simulink model "RALFMain"  (R2020a)
settings: Solver=FixedStepAuto  StartTime=0.0  StopTime=inf  FixedStep=0.01  RelTol=1e-3
InitFcn:
  | init
StopFcn:
  | stop
model workspace (MAT data in the model file):
  SL_ROS_VariableLengthArrays_MaxSizes.CommonInfo.ArrayTruncateAction = 'EmitWarning'
  SL_ROS_VariableLengthArrays_MaxSizes.MsgTypeMap = containers.Map
  SL_ROS_VariableLengthArrays_MaxSizes.MsgTypeMap.serialization.keys = {'sensor_msgs/Joy', 'std_msgs/Float32MultiArray', 'std_msgs/Int16MultiArray', 'std_msgs/Int32MultiArray', 'std_msgs/UInt16MultiArray', 'std_msgs/UInt8MultiArray'}
  SL_ROS_VariableLengthArrays_MaxSizes.MsgTypeMap.serialization.values{1}(1).PropertyName = 'Axes'
  SL_ROS_VariableLengthArrays_MaxSizes.MsgTypeMap.serialization.values{1}(1).DataType = 'single'
  SL_ROS_VariableLengthArrays_MaxSizes.MsgTypeMap.serialization.values{1}(1).MaxLength = 8
  SL_ROS_VariableLengthArrays_MaxSizes.MsgTypeMap.serialization.values{1}(2).PropertyName = 'Buttons'
  SL_ROS_VariableLengthArrays_MaxSizes.MsgTypeMap.serialization.values{1}(2).DataType = 'int32'
  SL_ROS_VariableLengthArrays_MaxSizes.MsgTypeMap.serialization.values{1}(2).MaxLength = 15
  SL_ROS_VariableLengthArrays_MaxSizes.MsgTypeMap.serialization.values{2}.PropertyName = 'Data'
  SL_ROS_VariableLengthArrays_MaxSizes.MsgTypeMap.serialization.values{2}.DataType = 'single'
  SL_ROS_VariableLengthArrays_MaxSizes.MsgTypeMap.serialization.values{2}.MaxLength = 8
  SL_ROS_VariableLengthArrays_MaxSizes.MsgTypeMap.serialization.values{3}.PropertyName = 'Data'
  SL_ROS_VariableLengthArrays_MaxSizes.MsgTypeMap.serialization.values{3}.DataType = 'int16'
  SL_ROS_VariableLengthArrays_MaxSizes.MsgTypeMap.serialization.values{3}.MaxLength = 4
  SL_ROS_VariableLengthArrays_MaxSizes.MsgTypeMap.serialization.values{4}.PropertyName = 'Data'
  SL_ROS_VariableLengthArrays_MaxSizes.MsgTypeMap.serialization.values{4}.DataType = 'int32'
  SL_ROS_VariableLengthArrays_MaxSizes.MsgTypeMap.serialization.values{4}.MaxLength = 8
  SL_ROS_VariableLengthArrays_MaxSizes.MsgTypeMap.serialization.values{5}.PropertyName = 'Data'
  SL_ROS_VariableLengthArrays_MaxSizes.MsgTypeMap.serialization.values{5}.DataType = 'uint16'
  SL_ROS_VariableLengthArrays_MaxSizes.MsgTypeMap.serialization.values{5}.MaxLength = 8
  SL_ROS_VariableLengthArrays_MaxSizes.MsgTypeMap.serialization.values{6}.PropertyName = 'Data'
  SL_ROS_VariableLengthArrays_MaxSizes.MsgTypeMap.serialization.values{6}.DataType = 'uint8'
  SL_ROS_VariableLengthArrays_MaxSizes.MsgTypeMap.serialization.values{6}.MaxLength = 8
  SL_ROS_VariableLengthArrays_MaxSizes.MsgTypeMap.serialization.uniformity = 0
  SL_ROS_VariableLengthArrays_MaxSizes.MsgTypeMap.serialization.keyType = 'char'
  SL_ROS_VariableLengthArrays_MaxSizes.MsgTypeMap.serialization.valueType = 'any'
values from neighbouring files (symbols this model uses):
  nmax = 1000    [init.m]
  pwinkel = 1/20    (= 0.05)    [init.m]
  pwinkel_vel = -4    [init.m]
undefined symbols (not defined in the file or in its folder): Axes, Axes_SL_Info, Buttons, Buttons_SL_Info
libraries: simulink x13, robotlib x4, dspswit3 x4, robotcorelib x4, simulink_extras x3, aerolibutil x3, etargetslib x2, aerolibanimutils x1, sharedtransform x1
CloseFcn:
  | stop
settings Model: EnablePacing=on  Creator=alf  LastModifiedBy=alf
settings DataIOCC: ReturnWorkspaceOutputs=off
settings OptimizationCC: EnhancedBackFolding=on  PassReuseOutputArgsAs=Individual arguments  MaxStackSize=64  OptimizeBlockOrder=speed  DifferentSizesBufferReuse=on  OptimizationCustomize=off  EfficientTunableParamExpr=on
settings DebuggingCC: ParameterPrecisionLossMsg=none  ParameterTunabilityLossMsg=error  ArithmeticOperatorsInVariantConditions=warning
settings HardwareCC: ProdBitPerLong=64  ProdHWDeviceType=Intel->x86-64 (Linux 64)
settings SFSimCC: MATLABDynamicMemAlloc=off  CustomCodeUndefinedFunction=UseInterfaceOnly
settings RTWCC: SystemTargetFile=ert.tlc  HardwareBoard=Robot Operating System (ROS)  TemplateMakefile=ert_default_tmf  GenerateReport=on  Toolchain=Catkin  IncludeHyperlinkInReport=on  LaunchReport=on  TargetLang=C++  GenerateTraceInfo=on  GenerateTraceReport=on  GenerateTraceReportSl=on  GenerateTraceReportSf=on  GenerateTraceReportEml=on
settings CodeAppCC: ForceParamTrailComments=on  IgnoreCustomStorageClasses=off  OperatorAnnotations=on  SimulinkDataObjDesc=on  SFDataObjDesc=on  InsertBlockDesc=on
settings ERTTargetCC: SupportContinuousTime=on  SupportNonInlinedSFcns=on

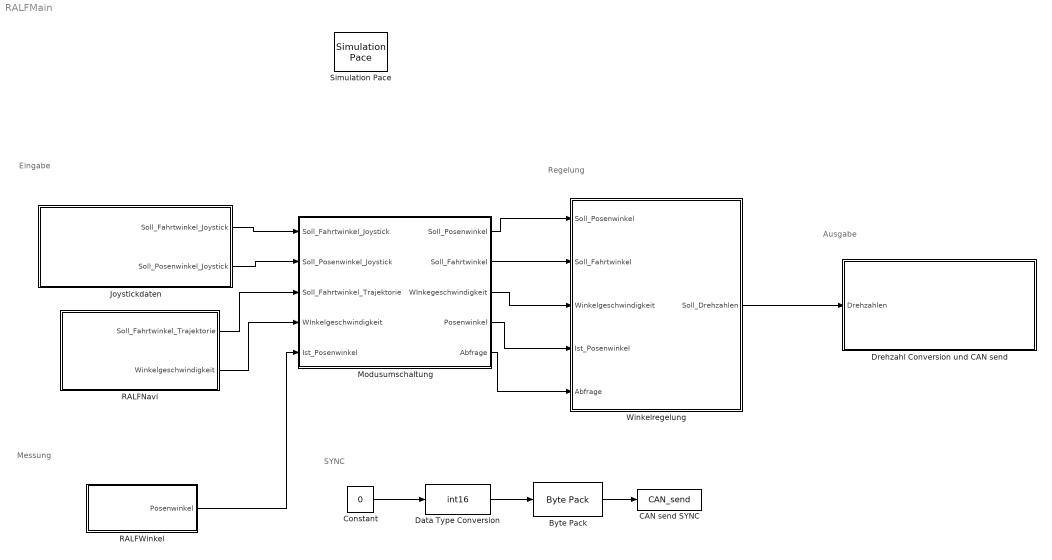
== system RALFMain ==
  note: SYNC
  note: Ausgabe
  note: Eingabe
  note: Messung
  note: Regelung
  Byte Pack : etargetslib/Byte Pack  datatypes={'int16'}  byteAlign=1
  CAN send SYNC : S-Function  FunctionName=CAN_send  Parameters=Port,Identifier  SFunctionModules=socketcan  SFunctionDeploymentMode=off  EnableBusSupport=off  mask{Port=can0, Identifier=hex2dec('80')}
      mask prompts: Port "CAN Port"
      mask TypeOptions Port: can0 | can1 | can2
      mask DialogControl DescTextVar Prompt: Dennis Hotze, Dominik Eickmann
  Constant : Constant  Value=0
  Data Type Conversion : DataTypeConversion  OutDataTypeStr=int16
  Drehzahl Conversion und CAN send : Subsystem
  Joystickdaten : Subsystem
  Modusumschaltung : Subsystem
  RALFNavi : Subsystem
  RALFWinkel : Subsystem
  Simulation Pace : aerolibanimutils/Simulation Pace  SimulationPace=1  SleepMode=Auto  OutputPaceError=off  SampleTime=-1
  Winkelregelung : Subsystem
  wires:
  Modusumschaltung/1(Soll_Posenwinkel) -> Winkelregelung/1(Soll_Posenwinkel)
  Modusumschaltung/2(Soll_Fahrtwinkel) -> Winkelregelung/2(Soll_Fahrtwinkel)
  Joystickdaten/1(Soll_Fahrtwinkel_Joystick) -> Modusumschaltung/1(Soll_Fahrtwinkel_Joystick)
  Joystickdaten/2(Soll_Posenwinkel_Joystick) -> Modusumschaltung/2(Soll_Posenwinkel_Joystick)
  Modusumschaltung/4(Posenwinkel) -> Winkelregelung/4(Ist_Posenwinkel)
  Modusumschaltung/3(WInkegeschwindigkeit) -> Winkelregelung/3(Winkelgeschwindigkeit)
  RALFWinkel/1(Posenwinkel) -> Modusumschaltung/5(Ist_Posenwinkel)
  RALFNavi/1(Soll_Fahrtwinkel_Trajektorie) -> Modusumschaltung/3(Soll_Fahrtwinkel_Trajektorie)
  RALFNavi/2("Winkelgeschwindigkeit ") -> Modusumschaltung/4("WInkelgeschwindigkeit ")
  Modusumschaltung/5(Abfrage) -> Winkelregelung/5("Abfrage ")
  Winkelregelung/1(Soll_Drehzahlen) -> Drehzahl Conversion und CAN send/1("Drehzahlen ")
  Data Type Conversion/1 -> Byte Pack/1
  Constant/1 -> Data Type Conversion/1
  Byte Pack/1 -> CAN send SYNC/1

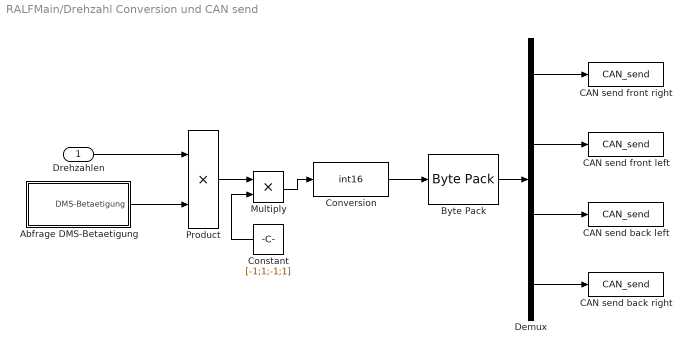
== system RALFMain/Drehzahl Conversion und CAN send ==
  "Drehzahlen " : Inport
  Abfrage DMS-Betaetigung : Subsystem
  Byte Pack : etargetslib/Byte Pack  datatypes={'int16'}  byteAlign=1
  CAN send back left : S-Function  FunctionName=CAN_send  Parameters=Port,Identifier  SFunctionModules=socketcan  SFunctionDeploymentMode=off  EnableBusSupport=off  mask{Port=can0, Identifier=hex2dec('121')}
      mask prompts: Port "CAN Port"
      mask TypeOptions Port: can0 | can1 | can2
      mask DialogControl DescTextVar Prompt: Dennis Hotze, Dominik Eickmann
  CAN send back right : S-Function  FunctionName=CAN_send  Parameters=Port,Identifier  SFunctionModules=socketcan  SFunctionDeploymentMode=off  EnableBusSupport=off  mask{Port=can0, Identifier=hex2dec('131')}
      mask prompts: Port "CAN Port"
      mask TypeOptions Port: can0 | can1 | can2
      mask DialogControl DescTextVar Prompt: Dennis Hotze, Dominik Eickmann
  CAN send front left : S-Function  FunctionName=CAN_send  Parameters=Port,Identifier  SFunctionModules=socketcan  SFunctionDeploymentMode=off  EnableBusSupport=off  mask{Port=can0, Identifier=hex2dec('111')}
      mask prompts: Port "CAN Port"
      mask TypeOptions Port: can0 | can1 | can2
      mask DialogControl DescTextVar Prompt: Dennis Hotze, Dominik Eickmann
  CAN send front right : S-Function  FunctionName=CAN_send  Parameters=Port,Identifier  SFunctionModules=socketcan  SFunctionDeploymentMode=off  EnableBusSupport=off  mask{Port=can0, Identifier=hex2dec('101')}
      mask prompts: Port "CAN Port"
      mask TypeOptions Port: can0 | can1 | can2
      mask DialogControl DescTextVar Prompt: Dennis Hotze, Dominik Eickmann
  Constant : Constant  Value=[-1;1;-1;1]
  "Conversion " : DataTypeConversion  OutDataTypeStr=int16
  Demux : Demux
  Multiply : Product
  Product : Product
  wires:
  "Drehzahlen "/1 -> Product/1
  Abfrage DMS-Betaetigung/1("DMS-Betaetigung ") -> Product/2
  "Conversion "/1 -> Byte Pack/1
  Demux/2 -> CAN send front left/1
  Byte Pack/1 -> Demux/1
  Demux/4 -> CAN send back right/1
  Demux/1 -> CAN send front right/1
  Demux/3 -> CAN send back left/1
  Product/1 -> Multiply/1
  Multiply/1 -> "Conversion "/1
  Constant/1 -> Multiply/2

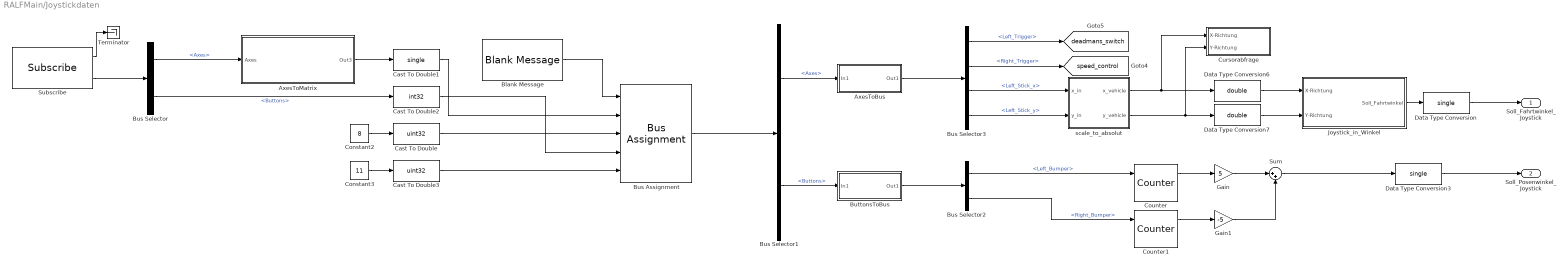
== system RALFMain/Joystickdaten ==
  AxesToBus : Subsystem
  AxesToMatrix : Subsystem
  Blank Message : robotlib/Blank Message  messageClass=Message  entityType=sensor_msgs/Joy  messageType=sensor_msgs/Joy  SampleTime=inf
  Bus Assignment : BusAssignment  AssignedSignals=Axes,Axes_SL_Info.CurrentLength,Buttons,Buttons_SL_Info.CurrentLength
  Bus Selector : BusSelector  OutputSignals=Axes,Buttons
  Bus Selector1 : BusSelector  OutputSignals=Axes,Buttons
  Bus Selector2 : BusSelector  OutputSignals=Bumper.Left_Bumper,Bumper.Right_Bumper
  Bus Selector3 : BusSelector  OutputSignals=Trigger.Left_Trigger,Trigger.Right_Trigger,Left_Stick.Left_Stick_x,Left_Stick.Left_Stick_y
  ButtonsToBus : Subsystem
  Cast To Double : DataTypeConversion  OutDataTypeStr=uint32
  Cast To Double1 : DataTypeConversion  OutDataTypeStr=single
  Cast To Double2 : DataTypeConversion  OutDataTypeStr=int32
  Cast To Double3 : DataTypeConversion  OutDataTypeStr=uint32
  Constant2 : Constant  Value=8
  Constant3 : Constant  Value=11
  Counter : dspswit3/Counter  Direction=Up  CountEvent=Rising edge  CounterSize=User defined  MaxCount=255  InitialCount=0  Output=Count and Hit  HitValue=32  ResetInput=on  SamplesPerFrame=1  Ts=1  CntDtype=double  HitDtype=Logical
  Counter1 : dspswit3/Counter  Direction=Up  CountEvent=Rising edge  CounterSize=User defined  MaxCount=255  InitialCount=0  Output=Count and Hit  HitValue=32  ResetInput=on  SamplesPerFrame=1  Ts=1  CntDtype=double  HitDtype=Logical
  Cursorabfrage : Subsystem
  Data Type Conversion : DataTypeConversion  OutDataTypeStr=single
  Data Type Conversion3 : DataTypeConversion  OutDataTypeStr=single
  Data Type Conversion6 : DataTypeConversion  OutDataTypeStr=double
  Data Type Conversion7 : DataTypeConversion  OutDataTypeStr=double
  Gain : Gain  Gain=5
  Gain1 : Gain  Gain=-5
  Joystick_in_Winkel : Subsystem
  Subscribe : robotlib/Subscribe  topicSource=Select from ROS network  topic=/joy  messageType=sensor_msgs/Joy  sampleTime=-1  messageQueueLength=1
  Sum : Sum  Inputs=|++
  Terminator : Terminator
  scale_to_absolut : Subsystem
  Soll_Fahrtwinkel_Joystick : Outport  VectorParamsAs1DForOutWhenUnconnected=off
  Soll_Posenwinkel_Joystick : Outport  Port=2  VectorParamsAs1DForOutWhenUnconnected=off
  tag scope: deadmans_switch=global, speed_control=global
  wires:
  Bus Selector2/2 -> Counter1/1  "<Right_Bumper>"
  Bus Selector2/1 -> Counter/1  "<Left_Bumper>"
  AxesToBus/1(Out1) -> Bus Selector3/1
  Bus Selector1/1 -> AxesToBus/1(In1)  "<Axes>"
  Bus Selector3/4 -> scale_to_absolut/2(y_in)  "<Left_Stick_y>"
  Bus Assignment/1 -> Bus Selector1/1
  ButtonsToBus/1(Out1) -> Bus Selector2/1
  Bus Selector3/3 -> scale_to_absolut/1(x_in)  "<Left_Stick_x>"
  Bus Selector1/2 -> ButtonsToBus/1(In1)  "<Buttons>"
  Bus Selector3/1 -> [deadmans_switch]  "<Left_Trigger>"
  scale_to_absolut/1(x_vehicle) -> Cursorabfrage/1(X-Richtung), Data Type Conversion6/1
  Data Type Conversion7/1 -> Joystick_in_Winkel/2(Y-Richtung)
  Data Type Conversion6/1 -> Joystick_in_Winkel/1(X-Richtung)
  Data Type Conversion/1 -> Soll_Fahrtwinkel_Joystick/1
  Joystick_in_Winkel/1(Soll_Fahrtwinkel) -> Data Type Conversion/1
  Data Type Conversion3/1 -> Soll_Posenwinkel_Joystick/1
  Sum/1 -> Data Type Conversion3/1
  scale_to_absolut/2(y_vehicle) -> Cursorabfrage/2(Y-Richtung), Data Type Conversion7/1
  Constant3/1 -> Cast To Double3/1
  Cast To Double1/1 -> Bus Assignment/2
  Blank Message/1 -> Bus Assignment/1
  AxesToMatrix/1(Out3) -> Cast To Double1/1
  Bus Selector/2 -> Cast To Double2/1  "<Buttons>"
  Constant2/1 -> Cast To Double/1
  Cast To Double/1 -> Bus Assignment/3
  Subscribe/2 -> Bus Selector/1
  Cast To Double2/1 -> Bus Assignment/4
  Subscribe/1 -> Terminator/1
  Bus Selector/1 -> AxesToMatrix/1(Axes)  "<Axes>"
  Cast To Double3/1 -> Bus Assignment/5
  Bus Selector3/2 -> [speed_control]  "<Right_Trigger>"
  Counter/1 -> Gain/1
  Gain/1 -> Sum/1
  Counter1/1 -> Gain1/1
  Gain1/1 -> Sum/2

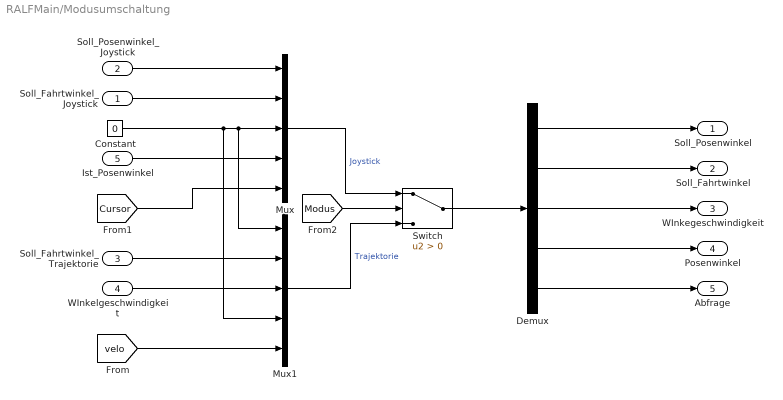
== system RALFMain/Modusumschaltung ==
  Soll_Fahrtwinkel_Joystick : Inport
  Soll_Posenwinkel_Joystick : Inport  Port=2
  Soll_Fahrtwinkel_Trajektorie : Inport  Port=3
  "WInkelgeschwindigkeit " : Inport  Port=4
  Ist_Posenwinkel : Inport  Port=5
  Constant : Constant  Value=0  OutDataTypeStr=single
  Demux : Demux  Outputs=5
  Mux : Mux  Inputs=5
  Mux1 : Mux  Inputs=5
  Switch : Switch  Criteria=u2 > Threshold
  Soll_Posenwinkel : Outport  VectorParamsAs1DForOutWhenUnconnected=off
  Soll_Fahrtwinkel : Outport  Port=2  VectorParamsAs1DForOutWhenUnconnected=off
  WInkegeschwindigkeit : Outport  Port=3  VectorParamsAs1DForOutWhenUnconnected=off
  Posenwinkel : Outport  Port=4  VectorParamsAs1DForOutWhenUnconnected=off
  Abfrage : Outport  Port=5  VectorParamsAs1DForOutWhenUnconnected=off
  wires:
  Switch/1 -> Demux/1
  Demux/2 -> Soll_Fahrtwinkel/1
  Demux/1 -> Soll_Posenwinkel/1
  Soll_Fahrtwinkel_Joystick/1 -> Mux/2
  Mux/1 -> Switch/1  "Joystick"
  Mux1/1 -> Switch/3  "Trajektorie"
  Constant/1 -> Mux1/4, Mux1/1, Mux/3
  Demux/3 -> WInkegeschwindigkeit/1
  Demux/4 -> Posenwinkel/1
  Soll_Posenwinkel_Joystick/1 -> Mux/1
  Ist_Posenwinkel/1 -> Mux/4
  Soll_Fahrtwinkel_Trajektorie/1 -> Mux1/2
  "WInkelgeschwindigkeit "/1 -> Mux1/3
  [Cursor] -> Mux/5
  [velo] -> Mux1/5
  Demux/5 -> Abfrage/1
  [Modus] -> Switch/2

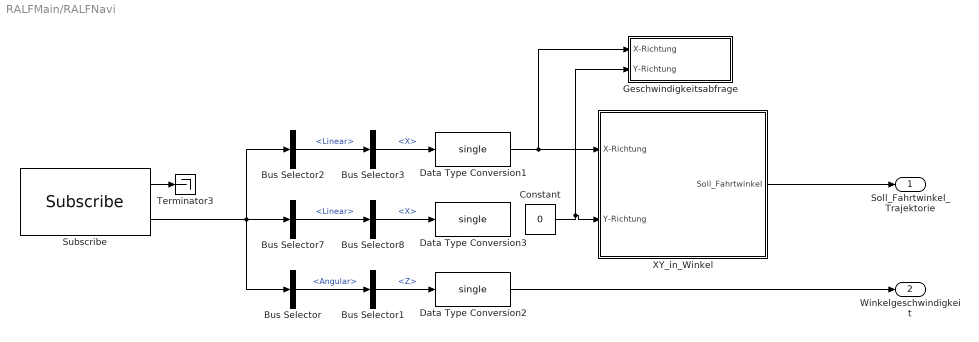
== system RALFMain/RALFNavi ==
  Bus Selector : BusSelector  OutputSignals=Angular
  Bus Selector1 : BusSelector  OutputSignals=Z
  Bus Selector2 : BusSelector  OutputSignals=Linear
  Bus Selector3 : BusSelector  OutputSignals=X
  Bus Selector7 : BusSelector  OutputSignals=Linear
  Bus Selector8 : BusSelector  OutputSignals=X
  Constant : Constant  Value=0  OutDataTypeStr=single
  Data Type Conversion1 : DataTypeConversion  OutDataTypeStr=single
  Data Type Conversion2 : DataTypeConversion  OutDataTypeStr=single
  Data Type Conversion3 : DataTypeConversion  OutDataTypeStr=single
  Geschwindigkeitsabfrage : Subsystem
  Subscribe : robotlib/Subscribe  topicSource=Select from ROS network  topic=/cmd_vel  messageType=geometry_msgs/Twist  sampleTime=-1  messageQueueLength=1
  Terminator3 : Terminator
  XY_in_Winkel : Subsystem
  Soll_Fahrtwinkel_Trajektorie : Outport  VectorParamsAs1DForOutWhenUnconnected=off
  "Winkelgeschwindigkeit " : Outport  Port=2  VectorParamsAs1DForOutWhenUnconnected=off
  wires:
  Bus Selector3/1 -> Data Type Conversion1/1  "<X>"
  Bus Selector2/1 -> Bus Selector3/1  "<Linear>"
  Bus Selector7/1 -> Bus Selector8/1  "<Linear>"
  Data Type Conversion2/1 -> "Winkelgeschwindigkeit "/1
  Bus Selector8/1 -> Data Type Conversion3/1  "<X>"
  Subscribe/2 -> Bus Selector7/1, Bus Selector/1, Bus Selector2/1
  Bus Selector1/1 -> Data Type Conversion2/1  "<Z>"
  Bus Selector/1 -> Bus Selector1/1  "<Angular>"
  Subscribe/1 -> Terminator3/1
  XY_in_Winkel/1(Soll_Fahrtwinkel) -> Soll_Fahrtwinkel_Trajektorie/1
  Data Type Conversion1/1 -> Geschwindigkeitsabfrage/1(X-Richtung), XY_in_Winkel/1(X-Richtung)
  Constant/1 -> Geschwindigkeitsabfrage/2(Y-Richtung), XY_in_Winkel/2(Y-Richtung)

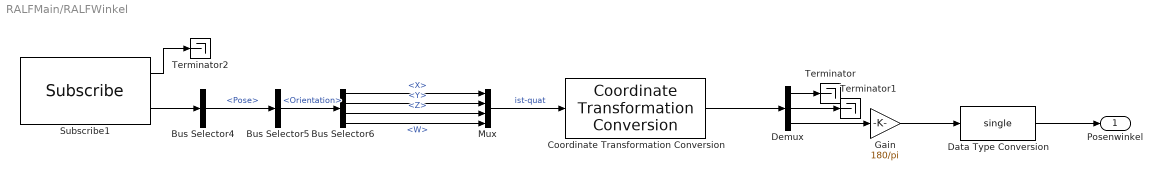
== system RALFMain/RALFWinkel ==
  Bus Selector4 : BusSelector  OutputSignals=Pose
  Bus Selector5 : BusSelector  OutputSignals=Orientation
  Bus Selector6 : BusSelector  OutputSignals=X,Y,Z,W
  Coordinate Transformation Conversion : robotcorelib/Coordinate Transformation Conversion  InputRepresentation=Quaternion  InputEulerSequence=ZYX  ShowTrVecInputPort=on  OutputRepresentation=Euler Angles  OutputEulerSequence=ZYX  ShowTrVecOutputPort=on  SimulateUsing=Interpreted execution
      settings: SourceProductBaseCode=NV,RO,RR
  Data Type Conversion : DataTypeConversion  OutDataTypeStr=single
  Demux : Demux  Outputs=3
  Gain : Gain  Gain=180/pi
  Mux : Mux
  Subscribe1 : robotlib/Subscribe  topicSource=Select from ROS network  topic=/slam_out_pose  messageType=geometry_msgs/PoseStamped  sampleTime=-1  messageQueueLength=1
  Terminator : Terminator
  Terminator1 : Terminator
  Terminator2 : Terminator
  Posenwinkel : Outport  VectorParamsAs1DForOutWhenUnconnected=off
  wires:
  Bus Selector6/4 -> Mux/4  "<W>"
  Bus Selector6/2 -> Mux/2  "<Y>"
  Bus Selector5/1 -> Bus Selector6/1  "<Orientation>"
  Bus Selector4/1 -> Bus Selector5/1  "<Pose>"
  Mux/1 -> Coordinate Transformation Conversion/1  "ist-quat"
  Subscribe1/2 -> Bus Selector4/1
  Bus Selector6/1 -> Mux/1  "<X>"
  Bus Selector6/3 -> Mux/3  "<Z>"
  Coordinate Transformation Conversion/1 -> Demux/1
  Demux/1 -> Terminator/1
  Demux/2 -> Terminator1/1
  Demux/3 -> Gain/1
  Subscribe1/1 -> Terminator2/1
  Gain/1 -> Data Type Conversion/1
  Data Type Conversion/1 -> Posenwinkel/1

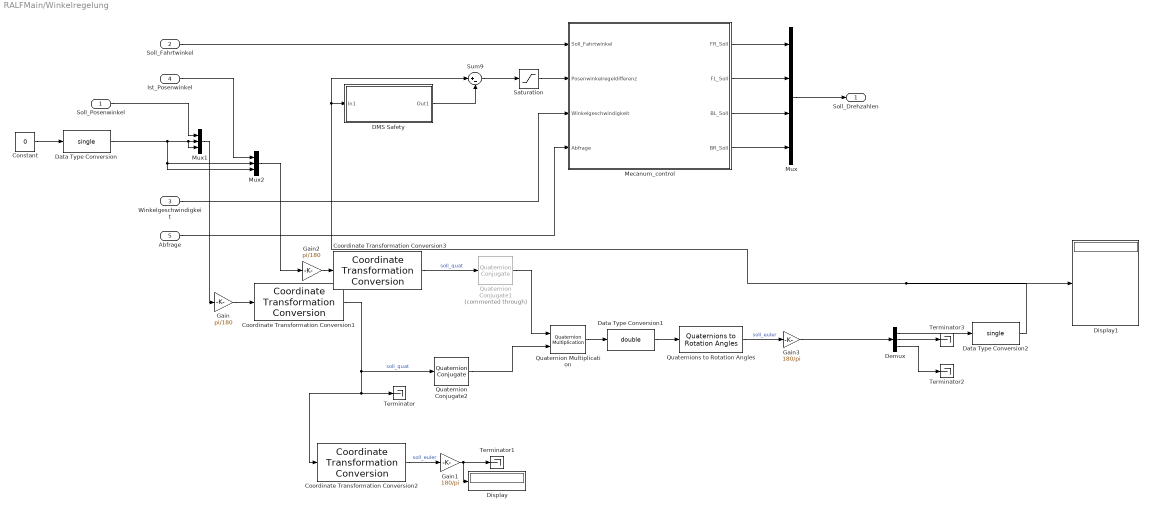
== system RALFMain/Winkelregelung ==
  Soll_Posenwinkel : Inport
  Soll_Fahrtwinkel : Inport  Port=2
  Winkelgeschwindigkeit : Inport  Port=3
  Ist_Posenwinkel : Inport  Port=4
  "Abfrage " : Inport  Port=5
  Constant : Constant  Value=0
  Coordinate Transformation Conversion1 : robotcorelib/Coordinate Transformation Conversion  InputRepresentation=Euler Angles  InputEulerSequence=ZYX  ShowTrVecInputPort=on  OutputRepresentation=Quaternion  OutputEulerSequence=ZYX  ShowTrVecOutputPort=on  SimulateUsing=Interpreted execution
      settings: SourceProductBaseCode=NV,RO,RR
  Coordinate Transformation Conversion2 : robotcorelib/Coordinate Transformation Conversion  InputRepresentation=Quaternion  InputEulerSequence=ZYX  ShowTrVecInputPort=on  OutputRepresentation=Euler Angles  OutputEulerSequence=ZYX  ShowTrVecOutputPort=on  SimulateUsing=Interpreted execution
      settings: SourceProductBaseCode=NV,RO,RR
  Coordinate Transformation Conversion3 : robotcorelib/Coordinate Transformation Conversion  InputRepresentation=Euler Angles  InputEulerSequence=ZYX  ShowTrVecInputPort=on  OutputRepresentation=Quaternion  OutputEulerSequence=ZYX  ShowTrVecOutputPort=on  SimulateUsing=Interpreted execution
      settings: SourceProductBaseCode=NV,RO,RR
  DMS Safety : Subsystem
  Data Type Conversion : DataTypeConversion  OutDataTypeStr=single
  Data Type Conversion1 : DataTypeConversion  OutDataTypeStr=double
  Data Type Conversion2 : DataTypeConversion  OutDataTypeStr=single
  Demux : Demux  Outputs=3
  Display : Display
  Display1 : Display
  Gain : Gain  Gain=pi/180
  Gain1 : Gain  Gain=180/pi
  Gain2 : Gain  Gain=pi/180
  Gain3 : Gain  Gain=180/pi
  Mecanum_control : Subsystem
  Mux : Mux
  Mux1 : Mux  Inputs=3
  Mux2 : Mux  Inputs=3
  Quaternion Conjugate1 : aerolibutil/Quaternion Conjugate  Commented=through
      settings: SourceProductBaseCode=AE
  Quaternion Conjugate2 : aerolibutil/Quaternion Conjugate
      settings: SourceProductBaseCode=AE
  Quaternion Multiplication : aerolibutil/Quaternion Multiplication
  Quaternions to Rotation Angles : sharedtransform/Quaternions to Rotation Angles  rotationOrder=ZYX  aMode=aMode
      settings: SourceProductBaseCode=AE,PW,MT,VE,VP
  Saturation : Saturate  UpperLimit=20  LowerLimit=-20
  Sum9 : Sum  Inputs=|+-
  Terminator{,1..3} (4 alike) : Terminator
  Soll_Drehzahlen : Outport  VectorParamsAs1DForOutWhenUnconnected=off
  wires:
  Soll_Posenwinkel/1 -> Mux1/1
  Soll_Fahrtwinkel/1 -> Mecanum_control/1(Soll_Fahrtwinkel)
  Sum9/1 -> Saturation/1
  Mecanum_control/1(FR_Soll) -> Mux/1
  Mecanum_control/4(BR_Soll) -> Mux/4
  Mecanum_control/2(FL_Soll) -> Mux/2
  Mecanum_control/3(BL_Soll) -> Mux/3
  Ist_Posenwinkel/1 -> Mux2/1
  Mux/1 -> Soll_Drehzahlen/1
  Winkelgeschwindigkeit/1 -> Mecanum_control/3(Winkelgeschwindigkeit)
  "Abfrage "/1 -> Mecanum_control/4(Abfrage)
  DMS Safety/1(Out1) -> Sum9/2
  Constant/1 -> Data Type Conversion/1
  Coordinate Transformation Conversion1/1 -> Quaternion Conjugate2/1, Coordinate Transformation Conversion2/1, Terminator/1  "soll_quat"
  Data Type Conversion/1 -> Mux2/3, Mux2/2, Mux1/3, Mux1/2
  Gain/1 -> Coordinate Transformation Conversion1/1
  Mux1/1 -> Gain/1
  Coordinate Transformation Conversion2/1 -> Gain1/1  "soll_euler"
  Gain1/1 -> Display/1, Terminator1/1
  Quaternion Multiplication/1 -> Data Type Conversion1/1
  Quaternions to Rotation Angles/1 -> Gain3/1  "soll_euler"
  Gain2/1 -> Coordinate Transformation Conversion3/1
  Coordinate Transformation Conversion3/1 -> Quaternion Conjugate1/1  "soll_quat"
  Mux2/1 -> Gain2/1
  Data Type Conversion1/1 -> Quaternions to Rotation Angles/1
  Quaternion Conjugate1/1 -> Quaternion Multiplication/1
  Demux/1 -> Data Type Conversion2/1
  Demux/3 -> Terminator2/1
  Demux/2 -> Terminator3/1
  Data Type Conversion2/1 -> Sum9/1, DMS Safety/1(In1), Display1/1
  Quaternion Conjugate2/1 -> Quaternion Multiplication/2
  Saturation/1 -> Mecanum_control/2(Posenwinkelregeldifferenz)
  Gain3/1 -> Demux/1

== system RALFMain/Drehzahl Conversion und CAN send/Abfrage DMS-Betaetigung ==
  Compare To Constant : simulink/Logic and Bit Operations/Compare To Constant  relop=>  const=0.9  OutDataTypeStr=boolean
  Data Type Conversion : DataTypeConversion  OutDataTypeStr=single
  "DMS-Betaetigung " : Outport  VectorParamsAs1DForOutWhenUnconnected=off
  wires:
  Compare To Constant/1 -> Data Type Conversion/1
  Data Type Conversion/1 -> "DMS-Betaetigung "/1
  [deadmans_switch] -> Compare To Constant/1

== system RALFMain/Joystickdaten/AxesToBus ==
  In1 : Inport
  Bus Creator{4..7} (4 alike) : BusCreator  Inputs=2
  Bus Creator8 : BusCreator  Inputs=4
  Demux : Demux  Outputs=8
  Out1 : Outport  VectorParamsAs1DForOutWhenUnconnected=off
  wires:
  Bus Creator4/1 -> Bus Creator8/1  "Left_Stick"
  Bus Creator5/1 -> Bus Creator8/3  "Right_Stick"
  Bus Creator6/1 -> Bus Creator8/2  "Trigger"
  Bus Creator7/1 -> Bus Creator8/4  "Direction_Pad"
  In1/1 -> Demux/1
  Demux/1 -> Bus Creator4/1  "Left_Stick_x"
  Demux/2 -> Bus Creator4/2  "Left_Stick_y"
  Demux/4 -> Bus Creator6/2  "Right_Trigger"
  Demux/3 -> Bus Creator6/1  "Left_Trigger"
  Demux/5 -> Bus Creator5/1  "Right_Stick_x"
  Demux/6 -> Bus Creator5/2  "Right_Stick_y"
  Demux/7 -> Bus Creator7/1  "Direction_Pad_x"
  Demux/8 -> Bus Creator7/2  "Direction_Pad_y"
  Bus Creator8/1 -> Out1/1

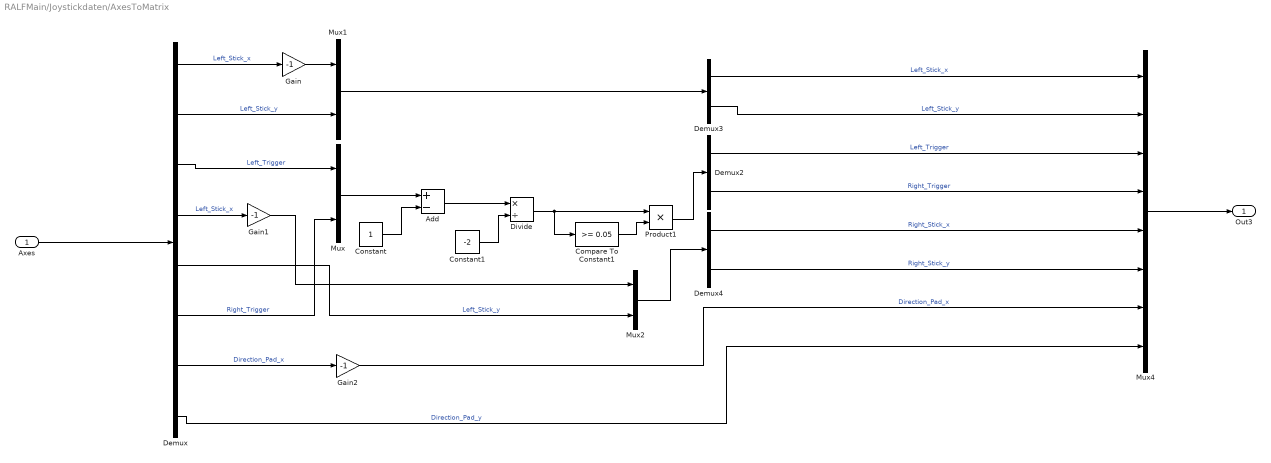
== system RALFMain/Joystickdaten/AxesToMatrix ==
  Axes : Inport
  Add : Sum  Inputs=+-
  Compare To Constant1 : simulink/Logic and Bit Operations/Compare To Constant  relop=>=  const=0.05  OutDataTypeStr=boolean
  Constant : Constant
  Constant1 : Constant  Value=-2
  Demux : Demux  Outputs=8
  Demux2 : Demux  Outputs=2
  Demux3 : Demux  Outputs=2
  Demux4 : Demux  Outputs=2
  Divide : Product  Inputs=*/
  Gain : Gain  Gain=-1
  Gain1 : Gain  Gain=-1
  Gain2 : Gain  Gain=-1
  Mux : Mux  Inputs=2
  Mux1 : Mux  Inputs=2
  Mux2 : Mux  Inputs=2
  Mux4 : Mux  Inputs=8
  Product1 : Product  OutDataTypeStr=single
  Out3 : Outport  VectorParamsAs1DForOutWhenUnconnected=off
  wires:
  Constant1/1 -> Divide/2
  Demux/5 -> Mux2/2  "Left_Stick_y"
  Demux/8 -> Mux4/8  "Direction_Pad_y"
  Mux/1 -> Add/1
  Demux/4 -> Gain1/1  "Left_Stick_x"
  Mux4/1 -> Out3/1
  Demux4/2 -> Mux4/6  "Right_Stick_y"
  Add/1 -> Divide/1
  Gain2/1 -> Mux4/7  "Direction_Pad_x"
  Demux/7 -> Gain2/1  "Direction_Pad_x"
  Demux3/1 -> Mux4/1  "Left_Stick_x"
  Demux/6 -> Mux/2  "Right_Trigger"
  Constant/1 -> Add/2
  Gain/1 -> Mux1/1
  Compare To Constant1/1 -> Product1/2
  Demux2/1 -> Mux4/3  "Left_Trigger"
  Divide/1 -> Compare To Constant1/1, Product1/1
  Product1/1 -> Demux2/1
  Demux3/2 -> Mux4/2  "Left_Stick_y"
  Demux2/2 -> Mux4/4  "Right_Trigger"
  Mux2/1 -> Demux4/1
  Demux4/1 -> Mux4/5  "Right_Stick_x"
  Axes/1 -> Demux/1
  Gain1/1 -> Mux2/1
  Demux/3 -> Mux/1  "Left_Trigger"
  Demux/1 -> Gain/1  "Left_Stick_x"
  Mux1/1 -> Demux3/1
  Demux/2 -> Mux1/2  "Left_Stick_y"

== system RALFMain/Joystickdaten/ButtonsToBus ==
  In1 : Inport
  Bus Creator : BusCreator  Inputs=6
  Bus Creator1 : BusCreator  Inputs=4
  Bus Creator2 : BusCreator  Inputs=2
  Bus Creator3 : BusCreator  Inputs=2
  Demux1 : Demux  Outputs=15
  Modusumschaltung : Subsystem
  Out1 : Outport  VectorParamsAs1DForOutWhenUnconnected=off
  wires:
  Demux1/9 -> Bus Creator/1  "XBOX_Guide_Button"
  Demux1/2 -> Modusumschaltung/1(B-Taste), Bus Creator1/2  "B"
  Demux1/11 -> Bus Creator3/2  "Right_Stick"
  Demux1/10 -> Bus Creator3/1  "Left_Stick"
  Bus Creator3/1 -> Bus Creator/6  "Sticks"
  Bus Creator1/1 -> Bus Creator/4  "ABXY"
  Demux1/1 -> Bus Creator1/1  "A"
  Bus Creator2/1 -> Bus Creator/5  "Bumper"
  Demux1/7 -> Bus Creator/3  "Back_Button"
  Demux1/4 -> Bus Creator1/4  "Y"
  Demux1/3 -> Bus Creator1/3  "X"
  Demux1/6 -> Bus Creator2/2  "Right_Bumper"
  Demux1/8 -> Bus Creator/2  "Start_Button"
  Demux1/5 -> Bus Creator2/1  "Left_Bumper"
  In1/1 -> Demux1/1
  Bus Creator/1 -> Out1/1

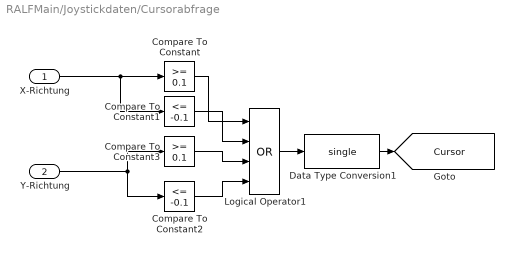
== system RALFMain/Joystickdaten/Cursorabfrage ==
  X-Richtung : Inport
  Y-Richtung : Inport  Port=2
  Compare To Constant : simulink/Logic and Bit Operations/Compare To Constant  relop=>=  const=0.1  OutDataTypeStr=boolean
  Compare To Constant1 : simulink/Logic and Bit Operations/Compare To Constant  relop=<=  const=-0.1  OutDataTypeStr=boolean
  Compare To Constant2 : simulink/Logic and Bit Operations/Compare To Constant  relop=<=  const=-0.1  OutDataTypeStr=boolean
  Compare To Constant3 : simulink/Logic and Bit Operations/Compare To Constant  relop=>=  const=0.1  OutDataTypeStr=boolean
  Data Type Conversion1 : DataTypeConversion  OutDataTypeStr=single
  Logical Operator1 : Logic  Operator=OR  Inputs=4  AllPortsSameDT=off  OutDataTypeStr=boolean
  tag scope: Cursor=global
  wires:
  X-Richtung/1 -> Compare To Constant1/1, Compare To Constant/1
  Y-Richtung/1 -> Compare To Constant3/1, Compare To Constant2/1
  Compare To Constant2/1 -> Logical Operator1/4
  Compare To Constant3/1 -> Logical Operator1/3
  Compare To Constant1/1 -> Logical Operator1/2
  Compare To Constant/1 -> Logical Operator1/1
  Logical Operator1/1 -> Data Type Conversion1/1
  Data Type Conversion1/1 -> [Cursor]

== system RALFMain/Joystickdaten/Joystick_in_Winkel ==
  X-Richtung : Inport
  Y-Richtung : Inport  Port=2
  Cartesian to Polar : simulink_extras/Transformations/Cartesian to Polar
  Soll_Fahrtwinkel : Outport  VectorParamsAs1DForOutWhenUnconnected=off
  wires:
  Cartesian to Polar/2 -> Soll_Fahrtwinkel/1
  X-Richtung/1 -> Cartesian to Polar/1
  Y-Richtung/1 -> Cartesian to Polar/2

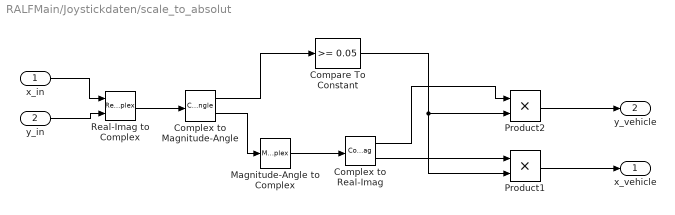
== system RALFMain/Joystickdaten/scale_to_absolut ==
  x_in : Inport
  y_in : Inport  Port=2
  Compare To Constant : simulink/Logic and Bit Operations/Compare To Constant  relop=>=  const=0.05  OutDataTypeStr=boolean
  Complex to Magnitude-Angle : ComplexToMagnitudeAngle
  Complex to Real-Imag : ComplexToRealImag
  Magnitude-Angle to Complex : MagnitudeAngleToComplex  Input=Angle  ConstantPart=1
  Product1 : Product
  Product2 : Product
  Real-Imag to Complex : RealImagToComplex
  x_vehicle : Outport  VectorParamsAs1DForOutWhenUnconnected=off
  y_vehicle : Outport  Port=2  VectorParamsAs1DForOutWhenUnconnected=off
  wires:
  Magnitude-Angle to Complex/1 -> Complex to Real-Imag/1
  Complex to Magnitude-Angle/2 -> Magnitude-Angle to Complex/1
  Product2/1 -> y_vehicle/1
  Compare To Constant/1 -> Product2/2, Product1/2
  Complex to Real-Imag/2 -> Product1/1
  Complex to Magnitude-Angle/1 -> Compare To Constant/1
  Real-Imag to Complex/1 -> Complex to Magnitude-Angle/1
  x_in/1 -> Real-Imag to Complex/1
  Complex to Real-Imag/1 -> Product2/1
  y_in/1 -> Real-Imag to Complex/2
  Product1/1 -> x_vehicle/1

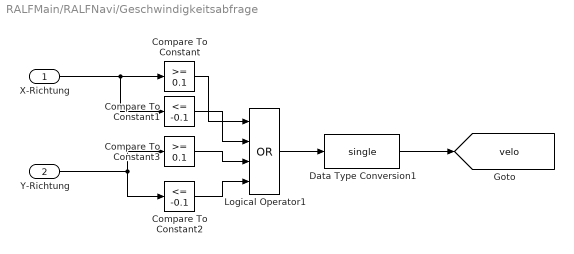
== system RALFMain/RALFNavi/Geschwindigkeitsabfrage ==
  X-Richtung : Inport
  Y-Richtung : Inport  Port=2
  Compare To Constant : simulink/Logic and Bit Operations/Compare To Constant  relop=>=  const=0.1  OutDataTypeStr=boolean
  Compare To Constant1 : simulink/Logic and Bit Operations/Compare To Constant  relop=<=  const=-0.1  OutDataTypeStr=boolean
  Compare To Constant2 : simulink/Logic and Bit Operations/Compare To Constant  relop=<=  const=-0.1  OutDataTypeStr=boolean
  Compare To Constant3 : simulink/Logic and Bit Operations/Compare To Constant  relop=>=  const=0.1  OutDataTypeStr=boolean
  Data Type Conversion1 : DataTypeConversion  OutDataTypeStr=single
  Logical Operator1 : Logic  Operator=OR  Inputs=4  AllPortsSameDT=off  OutDataTypeStr=boolean
  tag scope: velo=global
  wires:
  Compare To Constant3/1 -> Logical Operator1/3
  Compare To Constant2/1 -> Logical Operator1/4
  Compare To Constant/1 -> Logical Operator1/1
  Compare To Constant1/1 -> Logical Operator1/2
  Y-Richtung/1 -> Compare To Constant3/1, Compare To Constant2/1
  X-Richtung/1 -> Compare To Constant1/1, Compare To Constant/1
  Data Type Conversion1/1 -> [velo]
  Logical Operator1/1 -> Data Type Conversion1/1

== system RALFMain/RALFNavi/XY_in_Winkel ==
  X-Richtung : Inport
  Y-Richtung : Inport  Port=2
  Cartesian to Polar : simulink_extras/Transformations/Cartesian to Polar
  Soll_Fahrtwinkel : Outport  VectorParamsAs1DForOutWhenUnconnected=off
  wires:
  Cartesian to Polar/2 -> Soll_Fahrtwinkel/1
  X-Richtung/1 -> Cartesian to Polar/1
  Y-Richtung/1 -> Cartesian to Polar/2
  Cartesian to Polar/1 -> ?

== system RALFMain/Winkelregelung/DMS Safety ==
  In1 : Inport
  Abfrage DMS-Betaetigung : Subsystem
  Data Type Conversion : DataTypeConversion  OutDataTypeStr=single
  If Action Subsystem : Subsystem  TreatAsAtomicUnit=on
  Negation DMS : Subsystem
  Switch Case : SwitchCase
  Out1 : Outport  VectorParamsAs1DForOutWhenUnconnected=off
  wires:
  Negation DMS/1(DMS negiert) -> Data Type Conversion/1
  Data Type Conversion/1 -> Switch Case/1
  Switch Case/1 -> If Action Subsystem/Action
  In1/1 -> If Action Subsystem/1(In1)
  If Action Subsystem/1(Out1) -> Out1/1
  Abfrage DMS-Betaetigung/1("DMS-Betaetigung ") -> Negation DMS/1(DMS)

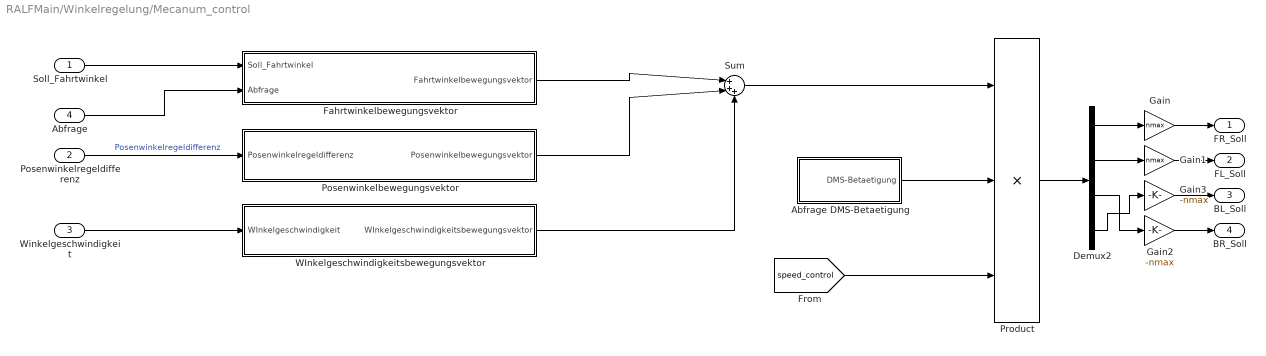
== system RALFMain/Winkelregelung/Mecanum_control ==
  Soll_Fahrtwinkel : Inport  OutDataTypeStr=single
  Posenwinkelregeldifferenz : Inport  Port=2  OutDataTypeStr=single
  Winkelgeschwindigkeit : Inport  Port=3  OutDataTypeStr=single
  Abfrage : Inport  Port=4  OutDataTypeStr=single
  Abfrage DMS-Betaetigung : Subsystem
  Demux2 : Demux
  Fahrtwinkelbewegungsvektor : Subsystem
  Gain : Gain  Gain=nmax  OutDataTypeStr=double
  Gain1 : Gain  Gain=nmax  OutDataTypeStr=double
  Gain2 : Gain  Gain=-nmax  OutDataTypeStr=double
  Gain3 : Gain  Gain=-nmax  OutDataTypeStr=double
  Posenwinkelbewegungsvektor : Subsystem
  Product : Product  Inputs=3  OutDataTypeStr=single
  Sum : Sum  Inputs=|+++
  WInkelgeschwindigkeitsbewegungsvektor : Subsystem
  FR_Soll : Outport  VectorParamsAs1DForOutWhenUnconnected=off
  FL_Soll : Outport  Port=2  VectorParamsAs1DForOutWhenUnconnected=off
  BL_Soll : Outport  Port=3  VectorParamsAs1DForOutWhenUnconnected=off
  BR_Soll : Outport  Port=4  VectorParamsAs1DForOutWhenUnconnected=off
  wires:
  Product/1 -> Demux2/1
  Demux2/2 -> Gain1/1
  Demux2/1 -> Gain/1
  Gain3/1 -> BL_Soll/1
  Gain2/1 -> BR_Soll/1
  Gain1/1 -> FL_Soll/1
  Gain/1 -> FR_Soll/1
  Demux2/3 -> Gain2/1
  Demux2/4 -> Gain3/1
  Fahrtwinkelbewegungsvektor/1(Fahrtwinkelbewegungsvektor) -> Sum/1
  Sum/1 -> Product/1
  Posenwinkelregeldifferenz/1 -> Posenwinkelbewegungsvektor/1(Posenwinkelregeldifferenz)  "Posenwinkelregeldifferenz"
  Soll_Fahrtwinkel/1 -> Fahrtwinkelbewegungsvektor/1(Soll_Fahrtwinkel)
  Winkelgeschwindigkeit/1 -> WInkelgeschwindigkeitsbewegungsvektor/1(WInkelgeschwindigkeit)
  WInkelgeschwindigkeitsbewegungsvektor/1("WInkelgeschwindigkeitsbewegungsvektor ") -> Sum/3
  Abfrage/1 -> Fahrtwinkelbewegungsvektor/2(Abfrage)
  Abfrage DMS-Betaetigung/1("DMS-Betaetigung ") -> Product/2
  [speed_control] -> Product/3
  Posenwinkelbewegungsvektor/1("Posenwinkelbewegungsvektor ") -> Sum/2

== system RALFMain/Joystickdaten/ButtonsToBus/Modusumschaltung ==
  B-Taste : Inport
  Constant : Constant  Value=2  OutDataTypeStr=single
  Counter : dspswit3/Counter  Direction=Up  CountEvent=Rising edge  CounterSize=User defined  MaxCount=255  InitialCount=0  Output=Count and Hit  HitValue=32  ResetInput=on  SamplesPerFrame=1  Ts=1  CntDtype=double  HitDtype=Logical
  Data Type Conversion : DataTypeConversion  OutDataTypeStr=single
  Data Type Conversion1 : DataTypeConversion  OutDataTypeStr=single
  Edge Detector : dspswit3/Edge Detector  InputProcessing=Columns as channels (frame based)
      settings: SourceProductBaseCode=DS
  Math Function : Math  Operator=mod  SignedPower=on  SaturateOnIntegerOverflow=on
  tag scope: Modus=global
  wires:
  B-Taste/1 -> Data Type Conversion/1
  Data Type Conversion1/1 -> Math Function/1
  Edge Detector/1 -> Counter/1
  Data Type Conversion/1 -> Edge Detector/1
  Constant/1 -> Math Function/2
  Counter/1 -> Data Type Conversion1/1
  Math Function/1 -> [Modus]

== system RALFMain/Winkelregelung/DMS Safety/Abfrage DMS-Betaetigung ==
  Compare To Constant : simulink/Logic and Bit Operations/Compare To Constant  relop=>  const=0.9  OutDataTypeStr=boolean
  Data Type Conversion : DataTypeConversion  OutDataTypeStr=single
  "DMS-Betaetigung " : Outport  VectorParamsAs1DForOutWhenUnconnected=off
  wires:
  Compare To Constant/1 -> Data Type Conversion/1
  Data Type Conversion/1 -> "DMS-Betaetigung "/1
  [deadmans_switch] -> Compare To Constant/1

== system RALFMain/Winkelregelung/DMS Safety/If Action Subsystem ==
  In1 : Inport
  Action Port : ActionPort  ActionPortLabel=case [ 1 ]:
  Out1 : Outport  VectorParamsAs1DForOutWhenUnconnected=off
  wires:
  In1/1 -> Out1/1

== system RALFMain/Winkelregelung/DMS Safety/Negation DMS ==
  DMS : Inport
  Constant : Constant  Value=-1
  Product1 : Product
  Sum4 : Sum  Inputs=|++
  DMS negiert : Outport  VectorParamsAs1DForOutWhenUnconnected=off
  wires:
  DMS/1 -> Sum4/1
  Constant/1 -> Product1/2, Sum4/2
  Sum4/1 -> Product1/1
  Product1/1 -> DMS negiert/1

== system RALFMain/Winkelregelung/Mecanum_control/Abfrage DMS-Betaetigung ==
  Compare To Constant : simulink/Logic and Bit Operations/Compare To Constant  relop=>  const=0.9  OutDataTypeStr=boolean
  Data Type Conversion : DataTypeConversion  OutDataTypeStr=single
  "DMS-Betaetigung " : Outport  VectorParamsAs1DForOutWhenUnconnected=off
  wires:
  Compare To Constant/1 -> Data Type Conversion/1
  Data Type Conversion/1 -> "DMS-Betaetigung "/1
  [deadmans_switch] -> Compare To Constant/1

== system RALFMain/Winkelregelung/Mecanum_control/Fahrtwinkelbewegungsvektor ==
  Soll_Fahrtwinkel : Inport
  Abfrage : Inport  Port=2
  Constant : Constant  Value=[1 -1;1 1;1 1;1 -1]  OutDataTypeStr=single
  Mux1 : Mux  Inputs=2
  Polar to Cartesian : simulink_extras/Transformations/Polar to Cartesian
      settings: SourceProductBaseCode=SL
  Product1 : Product  Multiplication=Matrix(*)
  Saturation3 : Saturate  UpperLimit=1  LowerLimit=-1
  Fahrtwinkelbewegungsvektor : Outport  VectorParamsAs1DForOutWhenUnconnected=off
  wires:
  Soll_Fahrtwinkel/1 -> Polar to Cartesian/2
  Polar to Cartesian/2 -> Mux1/2
  Constant/1 -> Product1/1
  Product1/1 -> Saturation3/1
  Abfrage/1 -> Polar to Cartesian/1
  Polar to Cartesian/1 -> Mux1/1
  Mux1/1 -> Product1/2
  Saturation3/1 -> Fahrtwinkelbewegungsvektor/1

== system RALFMain/Winkelregelung/Mecanum_control/Posenwinkelbewegungsvektor ==
  Posenwinkelregeldifferenz : Inport
  Constant1 : Constant  Value=[-1;1;-1;1]  OutDataTypeStr=single
  Gain4 : Gain  Gain=pwinkel
  Product2 : Product  Multiplication=Matrix(*)
  "Posenwinkelbewegungsvektor " : Outport  VectorParamsAs1DForOutWhenUnconnected=off
  wires:
  Constant1/1 -> Product2/1
  Gain4/1 -> Product2/2
  Product2/1 -> "Posenwinkelbewegungsvektor "/1
  Posenwinkelregeldifferenz/1 -> Gain4/1

== system RALFMain/Winkelregelung/Mecanum_control/WInkelgeschwindigkeitsbewegungsvektor ==
  WInkelgeschwindigkeit : Inport
  Constant1 : Constant  Value=[-1;1;-1;1]  OutDataTypeStr=single
  Gain4 : Gain  Gain=pwinkel_vel
  Product2 : Product  Multiplication=Matrix(*)
  "WInkelgeschwindigkeitsbewegungsvektor " : Outport  VectorParamsAs1DForOutWhenUnconnected=off
  wires:
  Constant1/1 -> Product2/1
  Gain4/1 -> Product2/2
  Product2/1 -> "WInkelgeschwindigkeitsbewegungsvektor "/1
  WInkelgeschwindigkeit/1 -> Gain4/1
